simulink model "Perception"  (R2024b)
settings: Solver=FixedStepAuto  StartTime=0.0  StopTime=10.0  RelTol=1e-3
undefined symbols (not defined in the file or in its folder): camera, gray
libraries: visionanalysis x6, visiongeotforms x1
settings Model: DataDictionary=DataDictionary.sldd  Creator=csamak  LastModifiedBy=tsamak
settings OptimizationCC: ZeroExternalMemoryAtStartup=off  ZeroInternalMemoryAtStartup=off  InitFltsAndDblsToZero=on
settings HardwareCC: ProdLongLongMode=on  TargetLongLongMode=on
settings SFSimCC: SimTargetLang=C++
settings RTWCC: TargetLang=C++  GenerateGPUCode=CUDA
settings GRTTargetCC: TargetLangStandard=C++11 (ISO)  CodeInterfacePackaging=C++ class

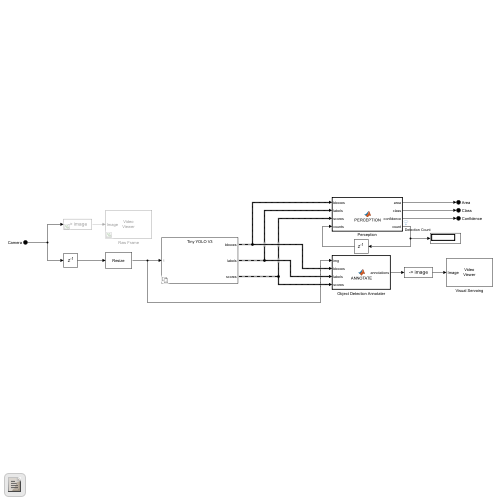
[thumbnail: Simulink's stored preview of the top-level diagram]
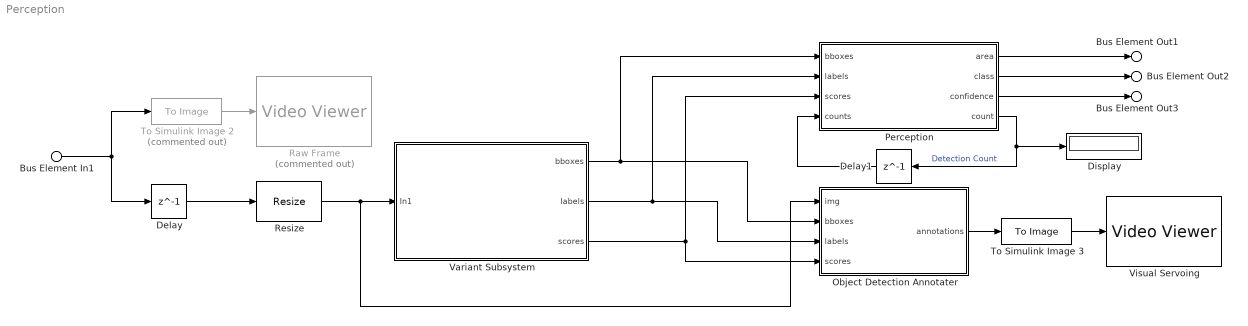
== system Perception ==
  Bus Element In1 : Inport  PortName=Camera
  Delay : Delay  DelayLength=1
  Delay1 : Delay  DelayLength=1
  Display : Display
  Object Detection Annotater : MATLAB Function  TreatAsAtomicUnit=on
  Perception : MATLAB Function  TreatAsAtomicUnit=on
  Raw Frame : VideoViewer  Commented=on  colormapValue=gray(256)  FigPos=[2.33333333333333 406.666666666667 418 304]
  Resize : visiongeotforms/Resize  specify=Number of output rows and columns  rfactor=[200 150]  outCols=25  outRows=25  outRowsCols=[360 640]  interp_method=Bilinear  antialias=on  useROI=off  roiFlag=off  roundingMode=Nearest  overflowMode=on  prodOutputMode=Binary point scaling  prodOutputWordLength=32  prodOutputFracLength=10
  To Simulink Image 2 : ToImage  Commented=on
  To Simulink Image 3 : ToImage
  Variant Subsystem : Subsystem  Variant=on  VariantActivationTime=inherit from Simulink.VariantControl
  Visual Servoing : VideoViewer  colormapValue=gray(256)  FigPos=[1177 538.666666666667 426 265.333333333333]
  Bus Element Out1 : Outport  PortName=Area
  Bus Element Out2 : Outport  Port=2  PortName=Class
  Bus Element Out3 : Outport  Port=3  PortName=Confidence
  wires:
  Delay/1 -> Resize/1
  To Simulink Image 2/1 -> Raw Frame/1
  Bus Element In1/1 -> To Simulink Image 2/1, Delay/1
  Resize/1 -> Variant Subsystem/1(In1), Object Detection Annotater/1(img)
  To Simulink Image 3/1 -> Visual Servoing/1
  Perception/3(confidence) -> Bus Element Out3/1
  Object Detection Annotater/1(annotations) -> To Simulink Image 3/1
  Perception/2(class) -> Bus Element Out2/1
  Perception/1(area) -> Bus Element Out1/1
  Variant Subsystem/1(bboxes) -> Object Detection Annotater/2(bboxes), Perception/1(bboxes)
  Variant Subsystem/2(labels) -> Object Detection Annotater/3(labels), Perception/2(labels)
  Variant Subsystem/3(scores) -> Object Detection Annotater/4(scores), Perception/3(scores)
  Perception/4(count) -> Delay1/1, Display/1  "Detection Count"
  Delay1/1 -> Perception/4(counts)

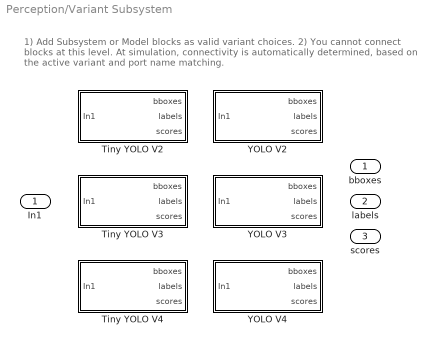
== system Perception/Variant Subsystem ==
  note: 1) Add Subsystem or Model blocks as valid variant choices.
      | 2) You cannot connect blocks at this level. At simulation, connectivity is automatically determined, based on the active variant and port name matching.
  In1 : Inport
  Tiny YOLO V2 : Subsystem  VariantControl=PERCEIVER==1
  Tiny YOLO V3 : Subsystem  VariantControl=PERCEIVER==2
  Tiny YOLO V4 : Subsystem  VariantControl=PERCEIVER==3
  YOLO V2 : Subsystem  VariantControl=PERCEIVER==4
  YOLO V3 : Subsystem  VariantControl=PERCEIVER==5
  YOLO V4 : Subsystem  VariantControl=PERCEIVER==6
  bboxes : Outport
  labels : Outport  Port=2
  scores : Outport  Port=3

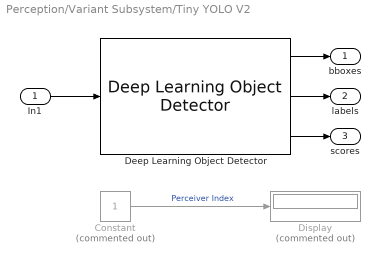
== system Perception/Variant Subsystem/Tiny YOLO V2 ==
  In1 : Inport
  Constant : Constant  Commented=on
  Deep Learning Object Detector : visionanalysis/Deep Learning Object Detector  Detector=Detector from MAT-file  DetectorFunction=vehicleDetectorYOLOv2  DetectorFilePath=yolov2_tiny.mat  MaxDetections=10  Bboxes=on  Scores=on  UseROI=off  AutoResize=on  ROI=[1 1 camera.ImageSize(2) round(camera.ImageSize(1)*0.678)]  Threshold=0.4  NumStrongestRegions=2000  UseMinSize=off  MinSize=[1 1]  UseMaxSize=off  MaxSize=[50 50]  ForceInterpretedSim=off
  Display : Display  Commented=on
  bboxes : Outport
  labels : Outport  Port=2
  scores : Outport  Port=3
  wires:
  In1/1 -> Deep Learning Object Detector/1
  Deep Learning Object Detector/2 -> labels/1
  Deep Learning Object Detector/1 -> bboxes/1
  Deep Learning Object Detector/3 -> scores/1
  Constant/1 -> Display/1  "Perceiver Index"

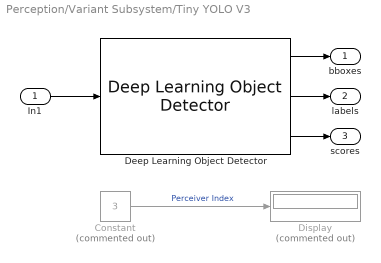
== system Perception/Variant Subsystem/Tiny YOLO V3 ==
  In1 : Inport
  Constant : Constant  Commented=on  Value=3
  Deep Learning Object Detector : visionanalysis/Deep Learning Object Detector  Detector=Detector from MAT-file  DetectorFunction=vehicleDetectorYOLOv2  DetectorFilePath=yolov3_tiny.mat  MaxDetections=10  Bboxes=on  Scores=on  UseROI=off  AutoResize=on  ROI=[1 1 camera.ImageSize(2) round(camera.ImageSize(1)*0.678)]  Threshold=0.4  NumStrongestRegions=2000  UseMinSize=off  MinSize=[1 1]  UseMaxSize=off  MaxSize=[50 50]  ForceInterpretedSim=off
  Display : Display  Commented=on
  bboxes : Outport
  labels : Outport  Port=2
  scores : Outport  Port=3
  wires:
  In1/1 -> Deep Learning Object Detector/1
  Deep Learning Object Detector/2 -> labels/1
  Deep Learning Object Detector/1 -> bboxes/1
  Deep Learning Object Detector/3 -> scores/1
  Constant/1 -> Display/1  "Perceiver Index"

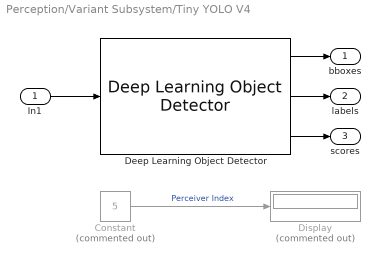
== system Perception/Variant Subsystem/Tiny YOLO V4 ==
  In1 : Inport
  Constant : Constant  Commented=on  Value=5
  Deep Learning Object Detector : visionanalysis/Deep Learning Object Detector  Detector=Detector from MAT-file  DetectorFunction=vehicleDetectorYOLOv2  DetectorFilePath=yolov4_tiny.mat  MaxDetections=10  Bboxes=on  Scores=on  UseROI=off  AutoResize=on  ROI=[1 1 camera.ImageSize(2) round(camera.ImageSize(1)*0.678)]  Threshold=0.4  NumStrongestRegions=2000  UseMinSize=off  MinSize=[1 1]  UseMaxSize=off  MaxSize=[50 50]  ForceInterpretedSim=off
  Display : Display  Commented=on
  bboxes : Outport
  labels : Outport  Port=2
  scores : Outport  Port=3
  wires:
  In1/1 -> Deep Learning Object Detector/1
  Deep Learning Object Detector/2 -> labels/1
  Deep Learning Object Detector/1 -> bboxes/1
  Deep Learning Object Detector/3 -> scores/1
  Constant/1 -> Display/1  "Perceiver Index"

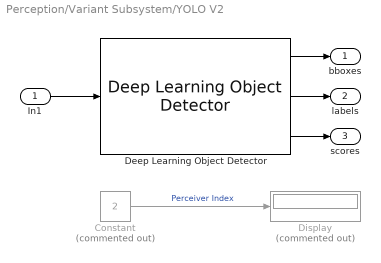
== system Perception/Variant Subsystem/YOLO V2 ==
  In1 : Inport
  Constant : Constant  Commented=on  Value=2
  Deep Learning Object Detector : visionanalysis/Deep Learning Object Detector  Detector=Detector from MAT-file  DetectorFunction=vehicleDetectorYOLOv2  DetectorFilePath=yolov2.mat  MaxDetections=10  Bboxes=on  Scores=on  UseROI=off  AutoResize=on  ROI=[1 1 camera.ImageSize(2) round(camera.ImageSize(1)*0.678)]  Threshold=0.4  NumStrongestRegions=2000  UseMinSize=off  MinSize=[1 1]  UseMaxSize=off  MaxSize=[50 50]  ForceInterpretedSim=off
  Display : Display  Commented=on
  bboxes : Outport
  labels : Outport  Port=2
  scores : Outport  Port=3
  wires:
  In1/1 -> Deep Learning Object Detector/1
  Deep Learning Object Detector/2 -> labels/1
  Deep Learning Object Detector/1 -> bboxes/1
  Deep Learning Object Detector/3 -> scores/1
  Constant/1 -> Display/1  "Perceiver Index"

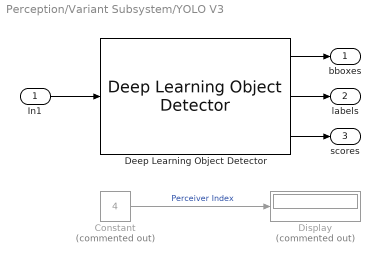
== system Perception/Variant Subsystem/YOLO V3 ==
  In1 : Inport
  Constant : Constant  Commented=on  Value=4
  Deep Learning Object Detector : visionanalysis/Deep Learning Object Detector  Detector=Detector from MAT-file  DetectorFunction=vehicleDetectorYOLOv2  DetectorFilePath=yolov3.mat  MaxDetections=10  Bboxes=on  Scores=on  UseROI=off  AutoResize=on  ROI=[1 1 camera.ImageSize(2) round(camera.ImageSize(1)*0.678)]  Threshold=0.4  NumStrongestRegions=2000  UseMinSize=off  MinSize=[1 1]  UseMaxSize=off  MaxSize=[50 50]  ForceInterpretedSim=off
  Display : Display  Commented=on
  bboxes : Outport
  labels : Outport  Port=2
  scores : Outport  Port=3
  wires:
  In1/1 -> Deep Learning Object Detector/1
  Deep Learning Object Detector/2 -> labels/1
  Deep Learning Object Detector/1 -> bboxes/1
  Deep Learning Object Detector/3 -> scores/1
  Constant/1 -> Display/1  "Perceiver Index"

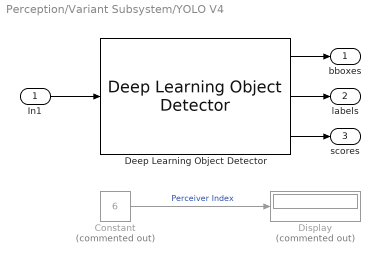
== system Perception/Variant Subsystem/YOLO V4 ==
  In1 : Inport
  Constant : Constant  Commented=on  Value=6
  Deep Learning Object Detector : visionanalysis/Deep Learning Object Detector  Detector=Detector from MAT-file  DetectorFunction=vehicleDetectorYOLOv2  DetectorFilePath=yolov4.mat  MaxDetections=10  Bboxes=on  Scores=on  UseROI=off  AutoResize=on  ROI=[1 1 camera.ImageSize(2) round(camera.ImageSize(1)*0.678)]  Threshold=0.4  NumStrongestRegions=2000  UseMinSize=off  MinSize=[1 1]  UseMaxSize=off  MaxSize=[50 50]  ForceInterpretedSim=off
  Display : Display  Commented=on
  bboxes : Outport
  labels : Outport  Port=2
  scores : Outport  Port=3
  wires:
  In1/1 -> Deep Learning Object Detector/1
  Deep Learning Object Detector/2 -> labels/1
  Deep Learning Object Detector/1 -> bboxes/1
  Deep Learning Object Detector/3 -> scores/1
  Constant/1 -> Display/1  "Perceiver Index"

== matlab function Perception/Perception ==
  data: bboxes input; area output; labels input; scores input; class output; confidence output; counts input; count output
function [area, class, confidence, count]= PERCEPTION(bboxes, labels, scores, counts)
    area = zeros(10,1);
    class = zeros(10,1);
    confidence = zeros(10,1);
    count = counts + size(bboxes,1);
    for i=1:size(bboxes,1)
        area(i) = bboxes(i,3)*bboxes(i,4);
        class(i) = labels(i);
        confidence(i) = scores(i);
    end

== matlab function Perception/Object Detection Annotater ==
  data: img input; annotations output; bboxes input; labels input; scores input
function annotations = ANNOTATE(img, bboxes, labels, scores)
    annotations = uint8(zeros(360,640,3));
    annotations = insertObjectAnnotation(img,"rectangle",bboxes,labels);
